simulink model "Elevator"  (R2023b)
settings: Solver=ode45  StartTime=0.0  StopTime=35  RelTol=1e-3
PreLoadFcn:
  | addpath(fullfile("ElevatorSupport","Scripts"));
  | addpath(fullfile("ElevatorSupport","Geometries"));
model workspace: external: MATLAB File Parameters.m (data not in the file)
undefined symbols (not defined in the file): BuildingTop, CabinFrame, CabinTopPlate, CounterWeight, CounterWeightFrame, CouterWeightRail, D, Door, DoorMechanismPlate, DoorPart, DoorStairOutTime1, DoorStairOutTime2, ElevatorCabin, ElevatorRail, Floor, FloorHeight, FloorStairOut, FloorTimeStairOut, g, K, MotorShaft, PrismaticJoint, Pulley, RevoluteJoint, RigidTransform, scale, Shaft, StairOutTime1, StairOutTime2, X, x, x2, Y, Z
libraries: sm_lib x283, nesl_utility x47
(part 1 of 6)
CloseFcn:
  | try
  |     close(fh);
  | catch
  | end
  | 
  | clear fh
  | clear logsoutElevator simlogElevator;
  | 
  | rmpath(fullfile("ElevatorSupport","Scripts"));
  | rmpath(fullfile("ElevatorSupport","Geometries"))
settings Model: Creator=The MathWorks, Inc.  LastModifiedBy=Aryasetya
settings SolverCC: AlgebraicLoopSolver=TrustRegion
settings DataIOCC: SaveTime=off  ReturnWorkspaceOutputs=off  SignalLoggingName=logsoutElevator
settings OptimizationCC: ReuseModelBlockBuffer=off
settings DebuggingCC: UnconnectedInputMsg=warning  UnconnectedOutputMsg=warning  UnconnectedLineMsg=warning  SubsystemReferenceDiagnosticForUnitTest=warning  SymbolicDimsDataTypeCodeGenerationDiagnostic=none
settings ModelReferenceCC: EnableRefExpFcnMdlSchedulingChecks=on
settings RTWCC: DLArmComputeVersion=19.05
settings SimscapeCC: SimscapeLogType=all  SimscapeLogSimulationStatistics=on  SimscapeLogName=simlogElevator  SimscapeLogLimitData=off
settings ExplorerConfigSet: InternalSimMechanicsExplorerSettings="<ExplorerConfiguration><canonicalview>default</canonicalview><AnimationSetting><BasePlaybackSpeed>1.0</BasePlaybackSpeed><PlaybackSpeedFactor>1.0</PlaybackSpeedFactor></AnimationSetting><TilePanel><TileInfo><Tiles Columns=\"2\" Count=\"2\" Rows=\"1\"><Column Weight=\"0.5\"/><Column Weight=\"0.5\"/><Row Weight=\"1\"/><Tile Height=\"1\" Width=\"1\" X=\"0\" Y=\"0\"/><Tile Height=\"1\" Width=\"1\" X=\"1\" Y=\"0\"/></Tiles></TileInfo><SceneInfo><SceneViewer><BGColor><R>1</R><G>1</G><B>1</B></BGColor><Camera><DoPerspective>off</DoPerspective><Position><X>20.7086531676557151</X><Y>-1.02984379292616524</Y><Z>-11.0864965005865486</Z></Position><Center><X>0.581530353759752927</X><Y>-1.02984379292616524</Y><Z>-11.0864965005865486</Z></Center><Up><X>-0</X><Y>0</Y><Z>1</Z></Up><ViewLimDist>1</ViewLimDist><YLim>16.4085643386840836</YLim><XLim>12.1235252438684942</XLim></Camera></SceneViewer><SceneViewer><BGColor><R>1</R><G>1</G><B>1</B></BGColor><Camera><DoPerspective>off</DoPerspective><Position><X>16.0519528198950141</X><Y>-9.70748669894142147</Y><Z>-4.07379558754266302</Z></Position><Center><X>-0.762288983658603869</X><Y>0.000137372139278557626</Y><Z>-12.8970022525360406</Z></Center><Up><X>-0.368402698741947754</X><Y>0.189189529780353194</Y><Z>0.910212488038446565</Z></Up><ViewLimDist>1</ViewLimDist><YLim>17.267396482909362</YLim><XLim>12.7580763822769807</XLim></Camera></SceneViewer></SceneInfo></TilePanel><MechEditorPanel><Cameras><Camera><Id>Camera1</Id><Value><Name>Camera1</Name><NativeCamera><PositionKeyframeSet><Keyframe><Time>+1.4390386105436841e+00</Time><Value><X>-1.9862962897423667e+01</X><Y>+3.7052197674734106e+00</Y><Z>+3.0536805221501222e+01</Z></Value></Keyframe><Keyframe><Time>+5.0767389598235519e+00</Time><Value><X>-4.7342144342170034e+00</X><Y>-1.0515849016541027e+01</Y><Z>+1.0916291278670778e+01</Z></Value></Keyframe><Keyframe><Time>+1.0381173794619109e+01</Time><Value><X>+1.3085629284472713e+00</X><Y>-1.0832577523234079e+01</Y><Z>+3.8731290903665652e+01</Z></Value></Keyframe><Keyframe><Time>+2.0000000000000000e+01</Time><Value><X>-1.9862962897423667e+01</X><Y>+3.7052197674734106e+00</Y><Z>+3.0536805221501222e+01</Z></Value></Keyframe></PositionKeyframeSet><CenterKeyframeSet><Keyframe><Time>+1.4390386105436841e+00</Time><Value><X>+2.3195990578990404e+00</X><Y>-1.1335086534382448e+01</Y><Z>+1.0722456628381920e+00</Z></Value></Keyframe><Keyframe><Time>+5.0767389598235519e+00</Time><Value><X>+1.2004004088622686e+00</X><Y>-1.4539659485468171e+01</Y><Z>+3.0334861791598531e+00</Z></Value></Keyframe><Keyframe><Time>+1.0381173794619109e+01</Time><Value><X>+1.3085629284472713e+00</X><Y>-1.0832577523234079e+01</Y><Z>+1.2891524079708603e+00</Z></Value></Keyframe><Keyframe><Time>+2.0000000000000000e+01</Time><Value><X>+2.3195990578990333e+00</X><Y>-1.1335086534382443e+01</Y><Z>+1.0722456628382027e+00</Z></Value></Keyframe></CenterKeyframeSet><UpVectorKeyframeSet><Keyframe><Time>+1.4390386105436841e+00</Time><Value><X>+2.1048840196857138e-01</X><Y>+9.2576466533046864e-01</Y><Z>-3.1409300702543935e-01</Z></Value></Keyframe><Keyframe><Time>+5.0767389598235519e+00</Time><Value><X>+2.1048840196857138e-01</X><Y>+9.2576466533046875e-01</Y><Z>-3.1409300702543930e-01</Z></Value></Keyframe><Keyframe><Time>+1.0381173794619109e+01</Time><Value><X>+0.0000000000000000e+00</X><Y>+1.0000000000000000e+00</Y><Z>-0.0000000000000000e+00</Z></Value></Keyframe><Keyframe><Time>+2.0000000000000000e+01</Time><Value><X>+2.1048840196857138e-01</X><Y>+9.2576466533046875e-01</Y><Z>-3.1409300702543935e-01</Z></Value></Keyframe></UpVectorKeyframeSet></NativeCamera></Value></Camera><Camera><Id>Camera2</Id><Value><Name>Camera2</Name><NativeCamera><PositionKeyframeSet/><CenterKeyframeSet/><UpVectorKeyframeSet/></NativeCamera></Value></Camera></Cameras><GfxPanelCameraMap/><VideoCreator><PlaybackSpeedRatio>1.0</PlaybackSpeedRatio><FrameRate>30</FrameRate><VideoFormat>Motion JPEG AVI</VideoFormat><FrameSize>auto</FrameSize></VideoCreator></MechEditorPanel></ExplorerConfiguration>"

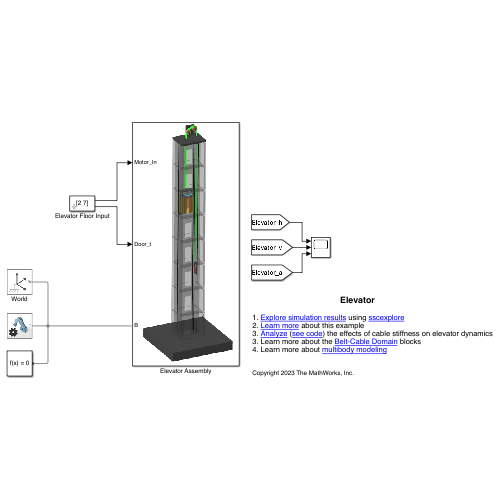
[thumbnail: Simulink's stored preview of the top-level diagram]
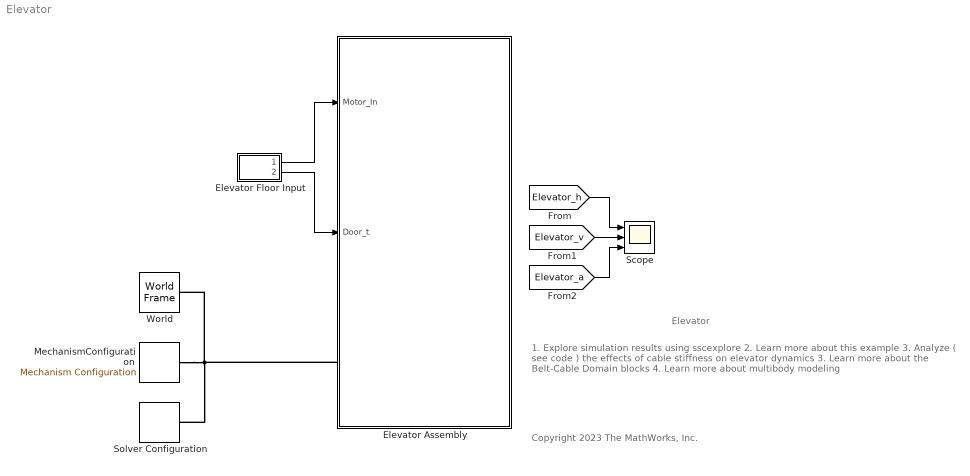
== system Elevator ==
  note: Copyright 2023 The MathWorks, Inc.
  note: 1. Explore simulation results using sscexplore
      | 2. Learn more about this example
      | 3. Analyze ( see code ) the effects of cable stiffness on elevator dynamics
      | 3. Learn more about the Belt-Cable Domain blocks
      | 4. Learn more about multibody modeling
  note: Elevator
  Elevator Assembly : Subsystem
      mask Display: image(fullfile('ElevatorSupport','Images','Full.png'));
  Elevator Floor Input : Subsystem  mask(Elevator Floors Input){FloorNums=[2 7]}
      mask prompts: FloorNums "Enter Floor Numbers"
      mask help:
      | Provide the floor numbers (1 to 7) for the elevator. This should be a (1 x n) vector. (n<=3)
      |
      | For example, an input of [4 2] means the elevator will go to the 4th Floor first and then the 2nd Floor.
      mask init:
      | if ~isrow(str2num(get_param(gcb,'FloorNums')))
      |     error('Input should be a row vector');
      | end
      | 
      | if length(str2num(get_param(gcb,'FloorNums')))>3
      |     error('Length of input row vector should not be greater then 3');
      | end
      | 
      | if any(str2num(get_param(gcb,'FloorNums'))>7)
      |     error('Elevator can not go above 7 floors for this system');
      | end
      | 
      | if any(str2num(get_param(gcb,'FloorNums'))<=0)
      |     error('Elevator floor input should be greater then 0');
      | end
      mask Display: disp(get_param(gcb,'FloorNums'));
  MechanismConfiguration : sm_lib/Utilities/Mechanism Configuration  UniformGravity=Constant  GravityVector=[0 0 -g]  GravityVectorUnits=m/s^2  LinearizationDelta=0.001  JointModeTransitionNonlinearIterations=2
  Scope : Scope  NumInputPorts=3
  Solver Configuration : nesl_utility/Solver Configuration  PhysicalDomain=network_engine_domain  SubClassName=solver  LeftPortType=input  RightPortType=generic  Tones=[]  Harmonics=[]  SimulateNoise=off  Profile=off  UseLocalSampling=off  EnableSwitchedLinearOptims=on  FrequencyDomain=off  UseCCode=off  RelTol=0.001  AbsTol=1e-06  MinStep=1e-09  ToWorkspace=off  RevertToSquareIcSolve=off  NumHomotopyIterations=100  PhasorMode=off  PhasorModeNumHarmonics=1  ConsistencySolver=NEWTON_FTOL  IndexReductionMethod=DerivativeReplacement  DoDC=off  ResidualTolerance=1e-09  ConsistencyTolSource=GLOBAL  ConsistencyAbsTol=0.001  ConsistencyRelTol=0.001  ConsistencyTolFactor=0.001  UseLocalSolver=off  LocalSolverChoice=NE_BACKWARD_EULER_ADVANCER  ResolveIndetEquations=on  FunctionEvalNumThread=1  LocalSolverSampleTime=0.001  DoFixedCost=off  MaxNonlinIter=3  MaxModeIter=2  ComputeImpulses=off  ImpulseIterations=1  LinearAlgebra=auto  LinearAlgebraNumThread=0  EquationFormulation=NE_TIME_EF  DelaysMemoryBudget=1024  AutomaticFiltering=on  FilteringTimeConstant=0.001  PartitionStorageMethod=AS_NEEDED  PartitionMemoryBudget=1024  PartitionMethod=ROBUST  MultibodyUseLocalSolver=off  MultibodyLocalSolverChoice=ODE1  MultibodyLocalSolverSampleTime=0.001
  World : sm_lib/Frames and Transforms/World Frame
  wires:
  Elevator Floor Input/1(MotorMotion) -> Elevator Assembly/1(Motor_In)
  Elevator Floor Input/2(DoorOperationTimes) -> Elevator Assembly/2(Door_t)
  [Elevator_h] -> Scope/1
  [Elevator_v] -> Scope/2
  [Elevator_a] -> Scope/3
  connections:
  MechanismConfiguration/RConn1 -- World/RConn1 -- Elevator Assembly/LConn1 -- Solver Configuration/RConn1

== system Elevator/Elevator Assembly ==
  Motor_In : Inport
  Door_t : Inport  Port=2
  Building : Subsystem
      mask Display: image(fullfile('ElevatorSupport','Images','Building.png'));
  CounterWeight : Subsystem
      mask Display: image(fullfile('ElevatorSupport','Images','CounterWeight.png'));
  CounterWeightPrismatic : Subsystem
  ElevatorCabin : Subsystem
      mask Display: image(fullfile('ElevatorSupport','Images','Cabin.png'));
  ElevatorPrismatic : Subsystem
  MotorPulley : Subsystem
      mask Display: image(fullfile('ElevatorSupport','Images','MotorPulley.png'));
  Rigid Transform : sm_lib/Frames and Transforms/Rigid Transform  TranslationMethod=None  TranslationStandardOffset=0  TranslationStandardOffsetUnits=m  TranslationStandardAxis=+Z  TranslationCartesianOffset=[0 0 0]  TranslationCartesianOffsetUnits=m  TranslationROffset=0  TranslationROffsetUnits=m  TranslationZOffset=0  TranslationZOffsetUnits=m  TranslationThetaOffset=0  TranslationThetaOffsetUnits=deg  RotationMethod=StandardAxis  RotationAngleUnits=deg  RotationStandardAxis=+Z  RotationAngle=-90  RotationArbitraryAxis=[0 0 1]  FollAlignAxisA=+Y  BaseAlignAxisA=-Y  FollAlignAxisB=+X  BaseAlignAxisB=-X  RotationSequenceAxes=FollowerAxes  RotationSequence=XYX  RotationSequenceAngles=[0 0 0]  RotationSequenceAnglesUnits=deg  RotationMatrix=[1 0 0; 0 1 0; 0 0 1]  Quaternion=[1 0 0 0]
  B : PMIOPort  Side=Left
  wires:
  Door_t/1 -> ElevatorCabin/1(door_t)
  ElevatorPrismatic/1(pos) -> ElevatorCabin/2(h)
  Motor_In/1 -> MotorPulley/1(Motor_In)
  connections:
  MotorPulley/RConn1 -- ElevatorCabin/LConn5
  MotorPulley/RConn6 -- CounterWeight/RConn5
  CounterWeight/RConn3 -- MotorPulley/RConn4
  Rigid Transform/LConn1 -- B/RConn1
  MotorPulley/RConn7 -- ElevatorCabin/LConn1
  MotorPulley/RConn10 -- ElevatorCabin/LConn4
  MotorPulley/RConn5 -- CounterWeight/RConn4
  ElevatorPrismatic/LConn1 -- Building/LConn2
  CounterWeight/LConn1 -- CounterWeightPrismatic/RConn1
  CounterWeight/RConn2 -- MotorPulley/RConn3
  MotorPulley/RConn9 -- ElevatorCabin/LConn3
  Building/LConn1 -- MotorPulley/LConn1
  MotorPulley/RConn2 -- CounterWeight/RConn1
  MotorPulley/RConn8 -- ElevatorCabin/LConn2
  ElevatorPrismatic/RConn1 -- ElevatorCabin/RConn1
  Building/RConn1 -- Rigid Transform/RConn1
  CounterWeightPrismatic/LConn1 -- Building/LConn3

== system Elevator/Elevator Floor Input ==
  Abs : Abs  SaturateOnIntegerOverflow=off
  Clock1 : Clock
  Clock3 : Clock
  Constant1 : Constant
  Constant2 : Constant  Value=1.5
  FloorChangesStairSignal : Subsystem  mask{FloorNums=FloorNums}
      mask prompts: FloorNums "Enter Floor Nums for Elevator"
      mask init:
      | [FloorStairOut,FloorTimeStairOut,StairOutTime1,StairOutTime2,DoorStairOutTime1,DoorStairOutTime2]...
      |  = getLookUpTableData(FloorNums);
  Gain : Gain  Gain=1/Pulley.radius
  Gain1 : Gain  Gain=FloorHeight
  Integrator1 : Integrator
  MATLAB Function : MATLAB Function  TreatAsAtomicUnit=on
  MotorDirection : Signum
  Product : Product
  Scope1 : Scope
  MotorMotion : Outport  VectorParamsAs1DForOutWhenUnconnected=off
  DoorOperationTimes : Outport  Port=2  VectorParamsAs1DForOutWhenUnconnected=off
  wires:
  FloorChangesStairSignal/3(DoorTimeChanges) -> DoorOperationTimes/1
  Abs/1 -> MATLAB Function/2(total_dis)
  FloorChangesStairSignal/1(FloorChanges) -> MotorDirection/1, Gain1/1
  FloorChangesStairSignal/2(TimeChanges) -> MATLAB Function/5(StepTime)
  Clock1/1 -> FloorChangesStairSignal/1(In1)
  MATLAB Function/1(v_t) -> Product/2
  Product/1 -> Integrator1/1
  MotorDirection/1 -> Product/1
  Gain/1 -> MotorMotion/1
  Gain1/1 -> Abs/1
  Clock3/1 -> MATLAB Function/1(t)
  Constant1/1 -> MATLAB Function/3(a)
  Constant2/1 -> MATLAB Function/4(v_const)
  Integrator1/1 -> Scope1/1, Gain/1

== system Elevator/Elevator Assembly/Building ==
  Floors : Subsystem
      mask Display: image(fullfile('ElevatorSupport','Images','Floor.png'));
  LongRail_1_RIGID : Subsystem
      mask Display: image(fullfile('ElevatorSupport','Images','Rails.png'));
  LongRail_2_RIGID : Subsystem
      mask Display: image(fullfile('ElevatorSupport','Images','Rails.png'));
  Planar : sm_lib/Joints/Planar Joint  JointMode=Normal  SenseConstraintForce=off  SenseConstraintForceX=off  SenseConstraintForceY=off  SenseConstraintForceZ=off  SenseConstraintTorque=off  SenseConstraintTorqueX=off  SenseConstraintTorqueY=off  SenseConstraintTorqueZ=off  SenseTotalForce=off  SenseTotalForceX=off  SenseTotalForceY=off  SenseTotalForceZ=off  SenseTotalTorque=off  SenseTotalTorqueX=off  SenseTotalTorqueY=off  SenseTotalTorqueZ=off  CompositeWrenchDir=FollowerOnBase  CompositeWrenchFrame=BaseFrame  PxEquilibriumPosition=0  PxEquilibriumPositionUnits=m  PxSpringStiffness=0  PxSpringStiffnessUnits=N/m  PxDampingCoefficient=0  PxDampingCoefficientUnits=N/(m/s)  PxTorqueActuationMode=NoTorque  PxMotionActuationMode=ComputedMotion  PxSensePosition=off  PxSenseVelocity=off  PxSenseAcceleration=off  PxSenseTorqueForce=off  PxSenseLowerLimitTorqueForce=off  PxSenseUpperLimitTorqueForce=off  PxLowerLimitSpecify=off  PxLowerLimitBound=-1  PxLowerLimitBoundUnits=m  PxLowerLimitStiffness=1e6  PxLowerLimitStiffnessUnits=N/m  PxLowerLimitDamping=1e3  PxLowerLimitDampingUnits=N/(m/s)  PxLowerLimitTransitionRegionWidth=1e-4  PxLowerLimitTransitionRegionWidthUnits=m  PxUpperLimitSpecify=off  PxUpperLimitBound=1  PxUpperLimitBoundUnits=m  PxUpperLimitStiffness=1e6  PxUpperLimitStiffnessUnits=N/m  PxUpperLimitDamping=1e3  PxUpperLimitDampingUnits=N/(m/s)  PxUpperLimitTransitionRegionWidth=1e-4  PxUpperLimitTransitionRegionWidthUnits=m  PxPositionTargetSpecify=off  PxPositionTargetPriority=High  PxPositionTargetValue=0  PxPositionTargetValueUnits=m  PxVelocityTargetSpecify=off  PxVelocityTargetPriority=High  PxVelocityTargetValue=0  PxVelocityTargetValueUnits=m/s  PyEquilibriumPosition=0  PyEquilibriumPositionUnits=m  PySpringStiffness=0  PySpringStiffnessUnits=N/m  PyDampingCoefficient=0  PyDampingCoefficientUnits=N/(m/s)  PyTorqueActuationMode=NoTorque  PyMotionActuationMode=ComputedMotion  PySensePosition=off  PySenseVelocity=off  PySenseAcceleration=off  PySenseTorqueForce=off  PySenseLowerLimitTorqueForce=off  PySenseUpperLimitTorqueForce=off  PyLowerLimitSpecify=off  PyLowerLimitBound=-1  PyLowerLimitBoundUnits=m  PyLowerLimitStiffness=1e6  PyLowerLimitStiffnessUnits=N/m  PyLowerLimitDamping=1e3  PyLowerLimitDampingUnits=N/(m/s)  PyLowerLimitTransitionRegionWidth=1e-4  PyLowerLimitTransitionRegionWidthUnits=m  PyUpperLimitSpecify=off  PyUpperLimitBound=1  PyUpperLimitBoundUnits=m  PyUpperLimitStiffness=1e6  PyUpperLimitStiffnessUnits=N/m  PyUpperLimitDamping=1e3  PyUpperLimitDampingUnits=N/(m/s)  PyUpperLimitTransitionRegionWidth=1e-4  PyUpperLimitTransitionRegionWidthUnits=m  PyPositionTargetSpecify=off  PyPositionTargetPriority=High  PyPositionTargetValue=0  PyPositionTargetValueUnits=m  PyVelocityTargetSpecify=off  PyVelocityTargetPriority=High  PyVelocityTargetValue=0  PyVelocityTargetValueUnits=m/s  RzEquilibriumPosition=0  RzEquilibriumPositionUnits=rad  RzSpringStiffness=0  RzSpringStiffnessUnits=N*m/rad  RzDampingCoefficient=0  RzDampingCoefficientUnits=N*m/(rad/s)  RzTorqueActuationMode=NoTorque  RzMotionActuationMode=ComputedMotion  RzSensePosition=off  RzSenseVelocity=off  RzSenseAcceleration=off  RzSenseTorqueForce=off  RzSenseLowerLimitTorqueForce=off  RzSenseUpperLimitTorqueForce=off  RzLowerLimitSpecify=off  RzLowerLimitBound=-90  RzLowerLimitBoundUnits=deg  RzLowerLimitStiffness=1e4  RzLowerLimitStiffnessUnits=N*m/deg  RzLowerLimitDamping=10  RzLowerLimitDampingUnits=N*m/(deg/s)  RzLowerLimitTransitionRegionWidth=0.1  RzLowerLimitTransitionRegionWidthUnits=deg  RzUpperLimitSpecify=off  RzUpperLimitBound=90  RzUpperLimitBoundUnits=deg  RzUpperLimitStiffness=1e4  RzUpperLimitStiffnessUnits=N*m/deg  RzUpperLimitDamping=10  RzUpperLimitDampingUnits=N*m/(deg/s)  RzUpperLimitTransitionRegionWidth=0.1  RzUpperLimitTransitionRegionWidthUnits=deg  RzPositionTargetSpecify=off  RzPositionTargetPriority=High  RzPositionTargetValue=0  RzPositionTargetValueUnits=deg  RzVelocityTargetSpecify=off  RzVelocityTargetPriority=High  RzVelocityTargetValue=0  RzVelocityTargetValueUnits=deg/s
  Prismatic : sm_lib/Joints/Prismatic Joint  JointMode=Normal  SenseConstraintForce=off  SenseConstraintForceX=off  SenseConstraintForceY=off  SenseConstraintForceZ=off  SenseConstraintTorque=off  SenseConstraintTorqueX=off  SenseConstraintTorqueY=off  SenseConstraintTorqueZ=off  SenseTotalForce=off  SenseTotalForceX=off  SenseTotalForceY=off  SenseTotalForceZ=off  SenseTotalTorque=off  SenseTotalTorqueX=off  SenseTotalTorqueY=off  SenseTotalTorqueZ=off  CompositeWrenchDir=FollowerOnBase  CompositeWrenchFrame=BaseFrame  EquilibriumPosition=0  EquilibriumPositionUnits=m  SpringStiffness=0  SpringStiffnessUnits=N/m  DampingCoefficient=0  DampingCoefficientUnits=N/(m/s)  TorqueActuationMode=NoTorque  MotionActuationMode=ComputedMotion  SensePosition=off  SenseVelocity=off  SenseAcceleration=off  SenseTorqueForce=off  SenseLowerLimitTorqueForce=off  SenseUpperLimitTorqueForce=off  LowerLimitSpecify=off  LowerLimitBound=-1  LowerLimitBoundUnits=m  LowerLimitStiffness=1e6  LowerLimitStiffnessUnits=N/m  LowerLimitDamping=1e3  LowerLimitDampingUnits=N/(m/s)  LowerLimitTransitionRegionWidth=1e-4  LowerLimitTransitionRegionWidthUnits=m  UpperLimitSpecify=off  UpperLimitBound=1  UpperLimitBoundUnits=m  UpperLimitStiffness=1e6  UpperLimitStiffnessUnits=N/m  UpperLimitDamping=1e3  UpperLimitDampingUnits=N/(m/s)  UpperLimitTransitionRegionWidth=1e-4  UpperLimitTransitionRegionWidthUnits=m  PositionTargetSpecify=on  PositionTargetPriority=Low  PositionTargetValue=PrismaticJoint(1).Pz.Pos  PositionTargetValueUnits=m  VelocityTargetSpecify=off  VelocityTargetPriority=High  VelocityTargetValue=0  VelocityTargetValueUnits=m/s
  Rail1 : Subsystem
      mask Display: image(fullfile('ElevatorSupport','Images','Rails.png'));
  Rail2 : Subsystem
      mask Display: image(fullfile('ElevatorSupport','Images','Rails.png'));
  F1 : PMIOPort  Side=Left
  B : PMIOPort  Port=2  Side=Right
  F2 : PMIOPort  Port=3  Side=Left
  F3 : PMIOPort  Port=4  Side=Left
  connections:
  Rail1/LConn2 -- Rail2/RConn1
  Rail1/LConn1 -- B/RConn1
  LongRail_1_RIGID/LConn2 -- LongRail_2_RIGID/LConn2
  Floors/RConn1 -- Rail2/LConn1
  Rail1/RConn1 -- Planar/LConn1
  LongRail_2_RIGID/LConn1 -- Planar/RConn1
  Rail1/RConn2 -- Prismatic/LConn1
  LongRail_1_RIGID/LConn3 -- Prismatic/RConn1
  F2/RConn1 -- Rail2/LConn2
  Floors/LConn1 -- F1/RConn1
  LongRail_1_RIGID/LConn1 -- F3/RConn1

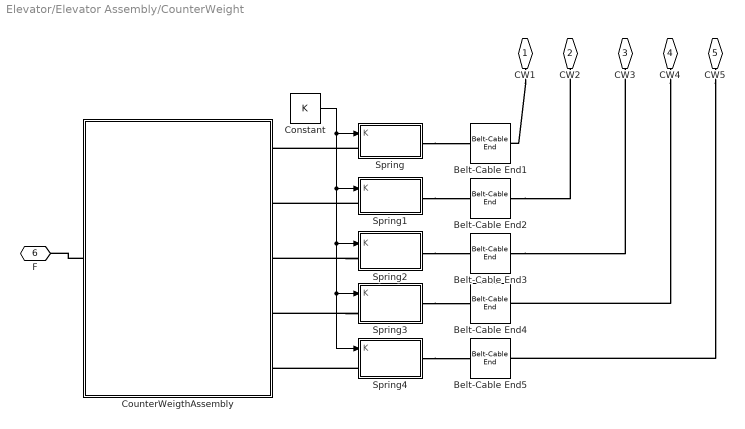
== system Elevator/Elevator Assembly/CounterWeight ==
  Belt-Cable End{1..5} (5 alike) : sm_lib/Belts and Cables/Belt-Cable End
  Constant : Constant  Value=K
  CounterWeigthAssembly : Subsystem
      mask Display: image(fullfile('ElevatorSupport','Images','CounterWeight.png'));
  Spring : Subsystem
  Spring1 : Subsystem
  Spring2 : Subsystem
  Spring3 : Subsystem
  Spring4 : Subsystem
  CW1 : PMIOPort  Side=Right
  CW2 : PMIOPort  Port=2  Side=Right
  CW3 : PMIOPort  Port=3  Side=Right
  CW4 : PMIOPort  Port=4  Side=Right
  CW5 : PMIOPort  Port=5  Side=Right
  F : PMIOPort  Port=6  Side=Left
  wires:
  Constant/1 -> Spring/1(K), Spring1/1(K), Spring2/1(K), Spring3/1(K), Spring4/1(K)
  connections:
  Spring3/RConn1 -- Belt-Cable End4/LConn1
  Spring2/RConn1 -- Belt-Cable End3/LConn1
  Spring2/LConn1 -- CounterWeigthAssembly/RConn3
  Spring4/LConn1 -- CounterWeigthAssembly/RConn5
  Spring/LConn1 -- CounterWeigthAssembly/RConn1
  Belt-Cable End2/RConn1 -- CW2/RConn1
  Spring1/LConn1 -- CounterWeigthAssembly/RConn2
  Spring1/RConn1 -- Belt-Cable End2/LConn1
  Belt-Cable End3/RConn1 -- CW3/RConn1
  CW1/RConn1 -- Belt-Cable End1/RConn1
  Spring4/RConn1 -- Belt-Cable End5/LConn1
  Spring3/LConn1 -- CounterWeigthAssembly/RConn4
  Spring/RConn1 -- Belt-Cable End1/LConn1
  CounterWeigthAssembly/LConn1 -- F/RConn1
  CW5/RConn1 -- Belt-Cable End5/RConn1
  CW4/RConn1 -- Belt-Cable End4/RConn1

== system Elevator/Elevator Assembly/CounterWeightPrismatic ==
  Prismatic Joint : sm_lib/Joints/Prismatic Joint  JointMode=Normal  SenseConstraintForce=off  SenseConstraintForceX=off  SenseConstraintForceY=off  SenseConstraintForceZ=off  SenseConstraintTorque=off  SenseConstraintTorqueX=off  SenseConstraintTorqueY=off  SenseConstraintTorqueZ=off  SenseTotalForce=off  SenseTotalForceX=off  SenseTotalForceY=off  SenseTotalForceZ=off  SenseTotalTorque=off  SenseTotalTorqueX=off  SenseTotalTorqueY=off  SenseTotalTorqueZ=off  CompositeWrenchDir=FollowerOnBase  CompositeWrenchFrame=BaseFrame  EquilibriumPosition=0  EquilibriumPositionUnits=m  SpringStiffness=0  SpringStiffnessUnits=N/m  DampingCoefficient=0  DampingCoefficientUnits=N/(m/s)  TorqueActuationMode=NoTorque  MotionActuationMode=ComputedMotion  SensePosition=off  SenseVelocity=off  SenseAcceleration=off  SenseTorqueForce=off  SenseLowerLimitTorqueForce=off  SenseUpperLimitTorqueForce=off  LowerLimitSpecify=off  LowerLimitBound=-1  LowerLimitBoundUnits=m  LowerLimitStiffness=1e6  LowerLimitStiffnessUnits=N/m  LowerLimitDamping=1e3  LowerLimitDampingUnits=N/(m/s)  LowerLimitTransitionRegionWidth=1e-4  LowerLimitTransitionRegionWidthUnits=m  UpperLimitSpecify=off  UpperLimitBound=1  UpperLimitBoundUnits=m  UpperLimitStiffness=1e6  UpperLimitStiffnessUnits=N/m  UpperLimitDamping=1e3  UpperLimitDampingUnits=N/(m/s)  UpperLimitTransitionRegionWidth=1e-4  UpperLimitTransitionRegionWidthUnits=m  PositionTargetSpecify=on  PositionTargetPriority=High  PositionTargetValue=7.5  PositionTargetValueUnits=m  VelocityTargetSpecify=off  VelocityTargetPriority=High  VelocityTargetValue=0  VelocityTargetValueUnits=m/s
  Rigid Transform : sm_lib/Frames and Transforms/Rigid Transform  TranslationMethod=None  TranslationStandardOffset=0  TranslationStandardOffsetUnits=m  TranslationStandardAxis=+Z  TranslationCartesianOffset=[0 0 0]  TranslationCartesianOffsetUnits=m  TranslationROffset=0  TranslationROffsetUnits=m  TranslationZOffset=0  TranslationZOffsetUnits=m  TranslationThetaOffset=0  TranslationThetaOffsetUnits=deg  RotationMethod=StandardAxis  RotationAngleUnits=deg  RotationStandardAxis=+Y  RotationAngle=90  RotationArbitraryAxis=[0 0 1]  FollAlignAxisA=+X  BaseAlignAxisA=+Y  FollAlignAxisB=+Y  BaseAlignAxisB=+Z  RotationSequenceAxes=FollowerAxes  RotationSequence=XYX  RotationSequenceAngles=[0 0 0]  RotationSequenceAnglesUnits=deg  RotationMatrix=[1 0 0; 0 1 0; 0 0 1]  Quaternion=[1 0 0 0]
  Rigid Transform1 : sm_lib/Frames and Transforms/Rigid Transform  TranslationMethod=None  TranslationStandardOffset=0  TranslationStandardOffsetUnits=m  TranslationStandardAxis=+Z  TranslationCartesianOffset=[0 0 0]  TranslationCartesianOffsetUnits=m  TranslationROffset=0  TranslationROffsetUnits=m  TranslationZOffset=0  TranslationZOffsetUnits=m  TranslationThetaOffset=0  TranslationThetaOffsetUnits=deg  RotationMethod=StandardAxis  RotationAngleUnits=deg  RotationStandardAxis=+Y  RotationAngle=-90  RotationArbitraryAxis=[0 0 1]  FollAlignAxisA=+X  BaseAlignAxisA=+Y  FollAlignAxisB=+Y  BaseAlignAxisB=+Z  RotationSequenceAxes=FollowerAxes  RotationSequence=XYX  RotationSequenceAngles=[0 0 0]  RotationSequenceAnglesUnits=deg  RotationMatrix=[1 0 0; 0 1 0; 0 0 1]  Quaternion=[1 0 0 0]
  B : PMIOPort  Side=Left
  F : PMIOPort  Port=2  Side=Right
  connections:
  Prismatic Joint/LConn1 -- Rigid Transform/RConn1
  Prismatic Joint/RConn1 -- Rigid Transform1/LConn1
  Rigid Transform1/RConn1 -- F/RConn1
  Rigid Transform/LConn1 -- B/RConn1

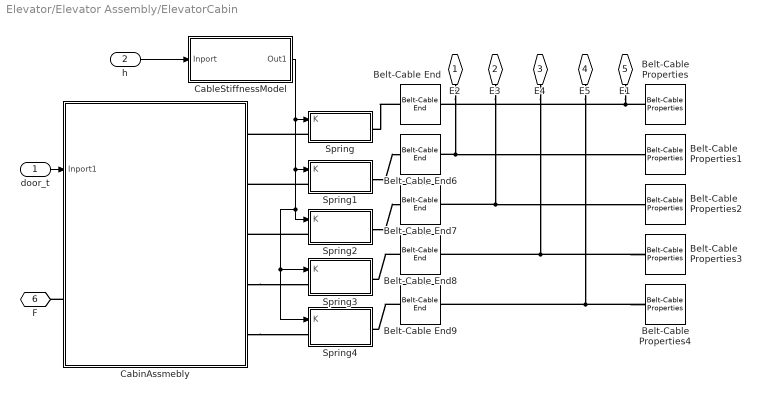
== system Elevator/Elevator Assembly/ElevatorCabin ==
  door_t : Inport
  h : Inport  Port=2
  Belt-Cable Properties{,1..4} (5 alike) : sm_lib/Belts and Cables/Belt-Cable Properties  DrumBeltCableAlignment=Unrestricted  GraphicType=PitchLine  GraphicVisPropType=SimpleVisualProperties  GraphicDiffuseColor=[0.2 1.0 0.2]  GraphicSpecularColor=[0.5 0.5 0.5 1.0]  GraphicAmbientColor=[0.15 0.15 0.15 1.0]  GraphicEmissiveColor=[0.0 0.0 0.0 1.0]  GraphicShininess=75  GraphicOpacity=1.0
  Belt-Cable End{,6..9} (5 alike) : sm_lib/Belts and Cables/Belt-Cable End
  CabinAssmebly : Subsystem
      mask Display: image(fullfile('ElevatorSupport','Images','CabinAssembly.png'));
  CableStiffnessModel : Subsystem  mask(Cable Stiffness){StiffnessModelChoice=Constant Stiffness}
      mask prompts: StiffnessModelChoice "StiffnessModel"
      mask help: Select Constant or Variable Stiffness values for approximating cable stiffness.
      mask TypeOptions StiffnessModelChoice: Constant Stiffness | Variable Stiffness
      mask Display: disp(get_param(gcb,'StiffnessModelChoice'))
  Spring : Subsystem
  Spring1 : Subsystem
  Spring2 : Subsystem
  Spring3 : Subsystem
  Spring4 : Subsystem
  E2 : PMIOPort  Side=Left
  E3 : PMIOPort  Port=2  Side=Left
  E4 : PMIOPort  Port=3  Side=Left
  E5 : PMIOPort  Port=4  Side=Left
  E1 : PMIOPort  Port=5  Side=Left
  F : PMIOPort  Port=6  Side=Right
  wires:
  door_t/1 -> CabinAssmebly/1(Inport1)
  CableStiffnessModel/1(Out1) -> Spring1/1(K), Spring4/1(K), Spring3/1(K), Spring2/1(K), Spring/1(K)
  h/1 -> CableStiffnessModel/1(Inport)
  connections:
  Belt-Cable Properties4/LConn1 -- Belt-Cable End9/RConn1 -- E5/RConn1
  CabinAssmebly/RConn5 -- Spring4/LConn1
  E3/RConn1 -- Belt-Cable End7/RConn1 -- Belt-Cable Properties2/LConn1
  Belt-Cable Properties3/LConn1 -- Belt-Cable End8/RConn1 -- E4/RConn1
  Spring2/RConn1 -- Belt-Cable End7/LConn1
  E2/RConn1 -- Belt-Cable Properties1/LConn1 -- Belt-Cable End6/RConn1
  Spring/LConn1 -- CabinAssmebly/RConn1
  Belt-Cable End8/LConn1 -- Spring3/RConn1
  Belt-Cable End/LConn1 -- Spring/RConn1
  Spring2/LConn1 -- CabinAssmebly/RConn3
  Belt-Cable End9/LConn1 -- Spring4/RConn1
  Spring1/LConn1 -- CabinAssmebly/RConn2
  Spring1/RConn1 -- Belt-Cable End6/LConn1
  CabinAssmebly/RConn4 -- Spring3/LConn1
  CabinAssmebly/LConn1 -- F/RConn1
  E1/RConn1 -- Belt-Cable Properties/LConn1 -- Belt-Cable End/RConn1

== system Elevator/Elevator Assembly/ElevatorPrismatic ==
  Abs : Abs  SaturateOnIntegerOverflow=off
  Add : Sum  Inputs=+-
  Constant : Constant  Value=-25.25
  PS-Simulink Converter : nesl_utility/PS-Simulink Converter  PhysicalDomain=network_engine_domain  SubClassName=ps_output  LeftPortType=input  RightPortType=output  PseudoPeriodic=off  Frequencies=[]  VectorFormat=1-D array  Unit=inherit  AffineConversion=off
  PS-Simulink Converter1 : nesl_utility/PS-Simulink Converter  PhysicalDomain=network_engine_domain  SubClassName=ps_output  LeftPortType=input  RightPortType=output  PseudoPeriodic=off  Frequencies=[]  VectorFormat=1-D array  Unit=inherit  AffineConversion=off
  PS-Simulink Converter2 : nesl_utility/PS-Simulink Converter  PhysicalDomain=network_engine_domain  SubClassName=ps_output  LeftPortType=input  RightPortType=output  PseudoPeriodic=off  Frequencies=[]  VectorFormat=1-D array  Unit=inherit  AffineConversion=off
  Prismatic Joint : sm_lib/Joints/Prismatic Joint  JointMode=Normal  SenseConstraintForce=off  SenseConstraintForceX=off  SenseConstraintForceY=off  SenseConstraintForceZ=off  SenseConstraintTorque=off  SenseConstraintTorqueX=off  SenseConstraintTorqueY=off  SenseConstraintTorqueZ=off  SenseTotalForce=off  SenseTotalForceX=off  SenseTotalForceY=off  SenseTotalForceZ=off  SenseTotalTorque=off  SenseTotalTorqueX=off  SenseTotalTorqueY=off  SenseTotalTorqueZ=off  CompositeWrenchDir=FollowerOnBase  CompositeWrenchFrame=BaseFrame  EquilibriumPosition=0  EquilibriumPositionUnits=m  SpringStiffness=0  SpringStiffnessUnits=N/m  DampingCoefficient=0  DampingCoefficientUnits=N/(m/s)  TorqueActuationMode=NoTorque  MotionActuationMode=ComputedMotion  SensePosition=on  SenseVelocity=on  SenseAcceleration=on  SenseTorqueForce=off  SenseLowerLimitTorqueForce=off  SenseUpperLimitTorqueForce=off  LowerLimitSpecify=off  LowerLimitBound=-1  LowerLimitBoundUnits=m  LowerLimitStiffness=1e6  LowerLimitStiffnessUnits=N/m  LowerLimitDamping=1e3  LowerLimitDampingUnits=N/(m/s)  LowerLimitTransitionRegionWidth=1e-4  LowerLimitTransitionRegionWidthUnits=m  UpperLimitSpecify=off  UpperLimitBound=1  UpperLimitBoundUnits=m  UpperLimitStiffness=1e6  UpperLimitStiffnessUnits=N/m  UpperLimitDamping=1e3  UpperLimitDampingUnits=N/(m/s)  UpperLimitTransitionRegionWidth=1e-4  UpperLimitTransitionRegionWidthUnits=m  PositionTargetSpecify=on  PositionTargetPriority=High  PositionTargetValue=-25.25  PositionTargetValueUnits=m  VelocityTargetSpecify=off  VelocityTargetPriority=Low  VelocityTargetValue=10  VelocityTargetValueUnits=m/s
  Rigid Transform : sm_lib/Frames and Transforms/Rigid Transform  TranslationMethod=None  TranslationStandardOffset=0  TranslationStandardOffsetUnits=m  TranslationStandardAxis=+Z  TranslationCartesianOffset=[0 0 0]  TranslationCartesianOffsetUnits=m  TranslationROffset=0  TranslationROffsetUnits=m  TranslationZOffset=0  TranslationZOffsetUnits=m  TranslationThetaOffset=0  TranslationThetaOffsetUnits=deg  RotationMethod=StandardAxis  RotationAngleUnits=deg  RotationStandardAxis=+Y  RotationAngle=90  RotationArbitraryAxis=[0 0 1]  FollAlignAxisA=+X  BaseAlignAxisA=+Y  FollAlignAxisB=+Y  BaseAlignAxisB=+Z  RotationSequenceAxes=FollowerAxes  RotationSequence=XYX  RotationSequenceAngles=[0 0 0]  RotationSequenceAnglesUnits=deg  RotationMatrix=[1 0 0; 0 1 0; 0 0 1]  Quaternion=[1 0 0 0]
  Rigid Transform1 : sm_lib/Frames and Transforms/Rigid Transform  TranslationMethod=None  TranslationStandardOffset=0  TranslationStandardOffsetUnits=m  TranslationStandardAxis=+Z  TranslationCartesianOffset=[0 0 0]  TranslationCartesianOffsetUnits=m  TranslationROffset=0  TranslationROffsetUnits=m  TranslationZOffset=0  TranslationZOffsetUnits=m  TranslationThetaOffset=0  TranslationThetaOffsetUnits=deg  RotationMethod=StandardAxis  RotationAngleUnits=deg  RotationStandardAxis=+Y  RotationAngle=-90  RotationArbitraryAxis=[0 0 1]  FollAlignAxisA=+X  BaseAlignAxisA=+Y  FollAlignAxisB=+Y  BaseAlignAxisB=+Z  RotationSequenceAxes=FollowerAxes  RotationSequence=XYX  RotationSequenceAngles=[0 0 0]  RotationSequenceAnglesUnits=deg  RotationMatrix=[1 0 0; 0 1 0; 0 0 1]  Quaternion=[1 0 0 0]
  F : PMIOPort  Side=Right
  B : PMIOPort  Port=2  Side=Left
  pos : Outport  VectorParamsAs1DForOutWhenUnconnected=off
  tag scope: Elevator_a=global, Elevator_h=global, Elevator_v=global
  wires:
  PS-Simulink Converter/1 -> Add/2, pos/1
  Add/1 -> Abs/1
  Constant/1 -> Add/1
  PS-Simulink Converter2/1 -> [Elevator_v]  "v"
  PS-Simulink Converter1/1 -> [Elevator_a]  "a"
  Abs/1 -> [Elevator_h]  "h"
  connections:
  Prismatic Joint/LConn1 -- Rigid Transform/RConn1
  Prismatic Joint/RConn1 -- Rigid Transform1/LConn1
  PS-Simulink Converter/LConn1 -- Prismatic Joint/RConn2
  Rigid Transform1/RConn1 -- F/RConn1
  Rigid Transform/LConn1 -- B/RConn1
  PS-Simulink Converter1/LConn1 -- Prismatic Joint/RConn4
  PS-Simulink Converter2/LConn1 -- Prismatic Joint/RConn3

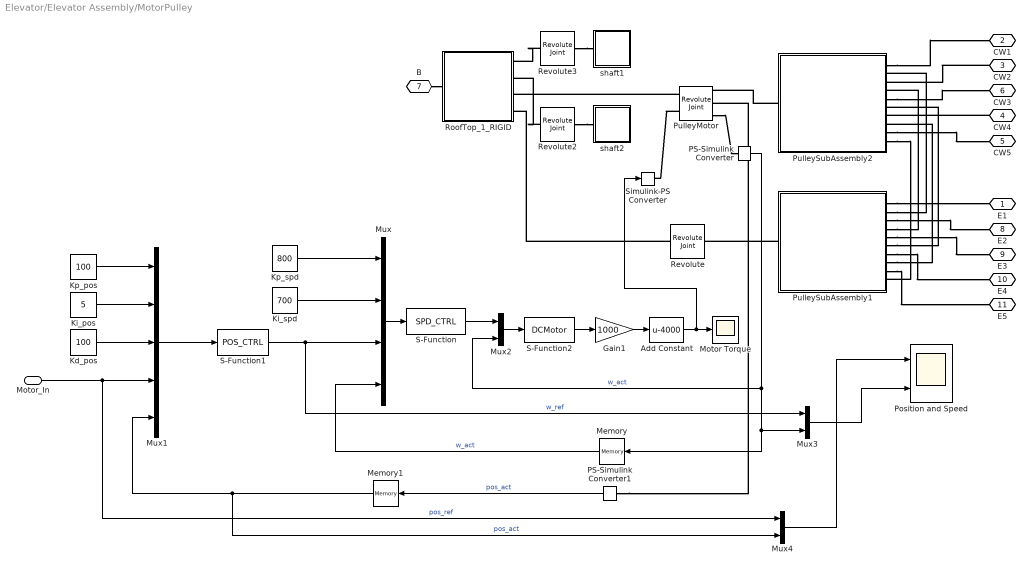
== system Elevator/Elevator Assembly/MotorPulley ==
  Motor_In : Inport
  Add Constant : Bias  Bias=-4000  SaturateOnIntegerOverflow=off
  Gain1 : Gain  Gain=1000
  Kd_pos : Constant  Value=100
  Ki_pos : Constant  Value=5
  Ki_spd : Constant  Value=700
  Kp_pos : Constant  Value=100
  Kp_spd : Constant  Value=800
  Memory : Memory
  Memory1 : Memory
  Motor Torque : Scope
  Mux : Mux
  Mux1 : Mux  Inputs=5
  Mux2 : Mux  Inputs=2
  Mux3 : Mux  Inputs=2
  Mux4 : Mux  Inputs=2
  PS-Simulink Converter : nesl_utility/PS-Simulink Converter  PhysicalDomain=network_engine_domain  SubClassName=ps_output  LeftPortType=input  RightPortType=output  PseudoPeriodic=off  Frequencies=[]  VectorFormat=inherit  Unit=inherit  AffineConversion=off
  PS-Simulink Converter1 : nesl_utility/PS-Simulink Converter  PhysicalDomain=network_engine_domain  SubClassName=ps_output  LeftPortType=input  RightPortType=output  PseudoPeriodic=off  Frequencies=[]  VectorFormat=inherit  Unit=inherit  AffineConversion=off
  Position and Speed : Scope  NumInputPorts=2
  PulleyMotor : sm_lib/Joints/Revolute Joint  JointMode=Normal  SenseConstraintForce=off  SenseConstraintForceX=off  SenseConstraintForceY=off  SenseConstraintForceZ=off  SenseConstraintTorque=off  SenseConstraintTorqueX=off  SenseConstraintTorqueY=off  SenseConstraintTorqueZ=off  SenseTotalForce=off  SenseTotalForceX=off  SenseTotalForceY=off  SenseTotalForceZ=off  SenseTotalTorque=off  SenseTotalTorqueX=off  SenseTotalTorqueY=off  SenseTotalTorqueZ=off  CompositeWrenchDir=FollowerOnBase  CompositeWrenchFrame=BaseFrame  EquilibriumPosition=0  EquilibriumPositionUnits=rad  SpringStiffness=0  SpringStiffnessUnits=N*m/rad  DampingCoefficient=0  DampingCoefficientUnits=N*m/(rad/s)  TorqueActuationMode=InputTorque  MotionActuationMode=ComputedMotion  SensePosition=on  SenseVelocity=on  SenseAcceleration=off  SenseTorqueForce=off  SenseLowerLimitTorqueForce=off  SenseUpperLimitTorqueForce=off  LowerLimitSpecify=off  LowerLimitBound=-90  LowerLimitBoundUnits=deg  LowerLimitStiffness=1e4  LowerLimitStiffnessUnits=N*m/deg  LowerLimitDamping=10  LowerLimitDampingUnits=N*m/(deg/s)  LowerLimitTransitionRegionWidth=0.1  LowerLimitTransitionRegionWidthUnits=deg  UpperLimitSpecify=off  UpperLimitBound=90  UpperLimitBoundUnits=deg  UpperLimitStiffness=1e4  UpperLimitStiffnessUnits=N*m/deg  UpperLimitDamping=10  UpperLimitDampingUnits=N*m/(deg/s)  UpperLimitTransitionRegionWidth=0.1  UpperLimitTransitionRegionWidthUnits=deg  PositionTargetSpecify=off  PositionTargetPriority=Low  PositionTargetValue=0  PositionTargetValueUnits=deg  VelocityTargetSpecify=off  VelocityTargetPriority=High  VelocityTargetValue=0  VelocityTargetValueUnits=deg/s
  PulleySubAssembly1 : Subsystem
      mask Display: image(fullfile('ElevatorSupport','Images','CabinPulley.png'));
  PulleySubAssembly2 : Subsystem
      mask Display: image(fullfile('ElevatorSupport','Images','CounterWeightPulley.png'));
  Revolute : sm_lib/Joints/Revolute Joint  JointMode=Normal  SenseConstraintForce=off  SenseConstraintForceX=off  SenseConstraintForceY=off  SenseConstraintForceZ=off  SenseConstraintTorque=off  SenseConstraintTorqueX=off  SenseConstraintTorqueY=off  SenseConstraintTorqueZ=off  SenseTotalForce=off  SenseTotalForceX=off  SenseTotalForceY=off  SenseTotalForceZ=off  SenseTotalTorque=off  SenseTotalTorqueX=off  SenseTotalTorqueY=off  SenseTotalTorqueZ=off  CompositeWrenchDir=FollowerOnBase  CompositeWrenchFrame=BaseFrame  EquilibriumPosition=0  EquilibriumPositionUnits=rad  SpringStiffness=0  SpringStiffnessUnits=N*m/rad  DampingCoefficient=0  DampingCoefficientUnits=N*m/(rad/s)  TorqueActuationMode=NoTorque  MotionActuationMode=ComputedMotion  SensePosition=off  SenseVelocity=off  SenseAcceleration=off  SenseTorqueForce=off  SenseLowerLimitTorqueForce=off  SenseUpperLimitTorqueForce=off  LowerLimitSpecify=off  LowerLimitBound=-90  LowerLimitBoundUnits=deg  LowerLimitStiffness=1e4  LowerLimitStiffnessUnits=N*m/deg  LowerLimitDamping=10  LowerLimitDampingUnits=N*m/(deg/s)  LowerLimitTransitionRegionWidth=0.1  LowerLimitTransitionRegionWidthUnits=deg  UpperLimitSpecify=off  UpperLimitBound=90  UpperLimitBoundUnits=deg  UpperLimitStiffness=1e4  UpperLimitStiffnessUnits=N*m/deg  UpperLimitDamping=10  UpperLimitDampingUnits=N*m/(deg/s)  UpperLimitTransitionRegionWidth=0.1  UpperLimitTransitionRegionWidthUnits=deg  PositionTargetSpecify=on  PositionTargetPriority=Low  PositionTargetValue=RevoluteJoint(1).Rz.Pos  PositionTargetValueUnits=deg  VelocityTargetSpecify=off  VelocityTargetPriority=High  VelocityTargetValue=1000  VelocityTargetValueUnits=deg/s
  Revolute2 : sm_lib/Joints/Revolute Joint  JointMode=Normal  SenseConstraintForce=off  SenseConstraintForceX=off  SenseConstraintForceY=off  SenseConstraintForceZ=off  SenseConstraintTorque=off  SenseConstraintTorqueX=off  SenseConstraintTorqueY=off  SenseConstraintTorqueZ=off  SenseTotalForce=off  SenseTotalForceX=off  SenseTotalForceY=off  SenseTotalForceZ=off  SenseTotalTorque=off  SenseTotalTorqueX=off  SenseTotalTorqueY=off  SenseTotalTorqueZ=off  CompositeWrenchDir=FollowerOnBase  CompositeWrenchFrame=BaseFrame  EquilibriumPosition=0  EquilibriumPositionUnits=rad  SpringStiffness=0  SpringStiffnessUnits=N*m/rad  DampingCoefficient=0  DampingCoefficientUnits=N*m/(rad/s)  TorqueActuationMode=NoTorque  MotionActuationMode=ComputedMotion  SensePosition=off  SenseVelocity=off  SenseAcceleration=off  SenseTorqueForce=off  SenseLowerLimitTorqueForce=off  SenseUpperLimitTorqueForce=off  LowerLimitSpecify=off  LowerLimitBound=-90  LowerLimitBoundUnits=deg  LowerLimitStiffness=1e4  LowerLimitStiffnessUnits=N*m/deg  LowerLimitDamping=10  LowerLimitDampingUnits=N*m/(deg/s)  LowerLimitTransitionRegionWidth=0.1  LowerLimitTransitionRegionWidthUnits=deg  UpperLimitSpecify=off  UpperLimitBound=90  UpperLimitBoundUnits=deg  UpperLimitStiffness=1e4  UpperLimitStiffnessUnits=N*m/deg  UpperLimitDamping=10  UpperLimitDampingUnits=N*m/(deg/s)  UpperLimitTransitionRegionWidth=0.1  UpperLimitTransitionRegionWidthUnits=deg  PositionTargetSpecify=on  PositionTargetPriority=Low  PositionTargetValue=RevoluteJoint(3).Rz.Pos  PositionTargetValueUnits=deg  VelocityTargetSpecify=off  VelocityTargetPriority=High  VelocityTargetValue=0  VelocityTargetValueUnits=deg/s
  Revolute3 : sm_lib/Joints/Revolute Joint  JointMode=Normal  SenseConstraintForce=off  SenseConstraintForceX=off  SenseConstraintForceY=off  SenseConstraintForceZ=off  SenseConstraintTorque=off  SenseConstraintTorqueX=off  SenseConstraintTorqueY=off  SenseConstraintTorqueZ=off  SenseTotalForce=off  SenseTotalForceX=off  SenseTotalForceY=off  SenseTotalForceZ=off  SenseTotalTorque=off  SenseTotalTorqueX=off  SenseTotalTorqueY=off  SenseTotalTorqueZ=off  CompositeWrenchDir=FollowerOnBase  CompositeWrenchFrame=BaseFrame  EquilibriumPosition=0  EquilibriumPositionUnits=rad  SpringStiffness=0  SpringStiffnessUnits=N*m/rad  DampingCoefficient=0  DampingCoefficientUnits=N*m/(rad/s)  TorqueActuationMode=NoTorque  MotionActuationMode=ComputedMotion  SensePosition=off  SenseVelocity=off  SenseAcceleration=off  SenseTorqueForce=off  SenseLowerLimitTorqueForce=off  SenseUpperLimitTorqueForce=off  LowerLimitSpecify=off  LowerLimitBound=-90  LowerLimitBoundUnits=deg  LowerLimitStiffness=1e4  LowerLimitStiffnessUnits=N*m/deg  LowerLimitDamping=10  LowerLimitDampingUnits=N*m/(deg/s)  LowerLimitTransitionRegionWidth=0.1  LowerLimitTransitionRegionWidthUnits=deg  UpperLimitSpecify=off  UpperLimitBound=90  UpperLimitBoundUnits=deg  UpperLimitStiffness=1e4  UpperLimitStiffnessUnits=N*m/deg  UpperLimitDamping=10  UpperLimitDampingUnits=N*m/(deg/s)  UpperLimitTransitionRegionWidth=0.1  UpperLimitTransitionRegionWidthUnits=deg  PositionTargetSpecify=on  PositionTargetPriority=Low  PositionTargetValue=RevoluteJoint(4).Rz.Pos  PositionTargetValueUnits=deg  VelocityTargetSpecify=off  VelocityTargetPriority=High  VelocityTargetValue=0  VelocityTargetValueUnits=deg/s
  RoofTop_1_RIGID : Subsystem
      mask Display: image(fullfile('ElevatorSupport','Images','Roof.png'));
  S-Function : S-Function  FunctionName=SPD_CTRL  SFunctionDeploymentMode=off  EnableBusSupport=off
  S-Function1 : S-Function  FunctionName=POS_CTRL  SFunctionDeploymentMode=off  EnableBusSupport=off
  S-Function2 : S-Function  FunctionName=DCMotor  SFunctionDeploymentMode=off  EnableBusSupport=off
  Simulink-PS Converter : nesl_utility/Simulink-PS Converter  PhysicalDomain=network_engine_domain  SubClassName=ps_input  LeftPortType=input  RightPortType=output  PseudoPeriodic=off  Frequencies=[]  NoiseDistribution=none  NoiseParameters=[]  Unit=1  AffineConversion=off  FilteringAndDerivatives=provide  SimscapeFilterOrder=1  InputFilterTimeConstant=0.001  UdotUserProvided=0
  shaft1 : Subsystem
  shaft2 : Subsystem
  E1 : PMIOPort  Side=Right
  CW1 : PMIOPort  Port=2  Side=Right
  CW2 : PMIOPort  Port=3  Side=Right
  CW4 : PMIOPort  Port=4  Side=Right
  CW5 : PMIOPort  Port=5  Side=Right
  CW3 : PMIOPort  Port=6  Side=Right
  B : PMIOPort  Port=7  Side=Left
  E2 : PMIOPort  Port=8  Side=Right
  E3 : PMIOPort  Port=9  Side=Right
  E4 : PMIOPort  Port=10  Side=Right
  E5 : PMIOPort  Port=11  Side=Right
  wires:
  Mux/1 -> S-Function/1
  Kp_spd/1 -> Mux/1
  Ki_spd/1 -> Mux/2
  PS-Simulink Converter/1 -> Mux3/2, Memory/1, Mux2/2  "w_act"
  Memory/1 -> Mux/4  "w_act"
  S-Function1/1 -> Mux3/1, Mux/3  "w_ref"
  Add Constant/1 -> Motor Torque/1, Simulink-PS Converter/1
  Mux1/1 -> S-Function1/1
  PS-Simulink Converter1/1 -> Memory1/1  "pos_act"
  Ki_pos/1 -> Mux1/2
  Kp_pos/1 -> Mux1/1
  Memory1/1 -> Mux4/2, Mux1/5  "pos_act"
  Motor_In/1 -> Mux4/1, Mux1/4  "pos_ref"
  S-Function/1 -> Mux2/1
  Mux2/1 -> S-Function2/1
  S-Function2/1 -> Gain1/1
  Gain1/1 -> Add Constant/1
  Kd_pos/1 -> Mux1/3
  Mux4/1 -> Position and Speed/1
  Mux3/1 -> Position and Speed/2
  connections:
  PulleySubAssembly1/RConn2 -- PulleySubAssembly2/RConn2
  Revolute3/LConn1 -- RoofTop_1_RIGID/RConn1
  PulleySubAssembly1/RConn4 -- PulleySubAssembly2/RConn4
  PulleySubAssembly1/RConn8 -- PulleySubAssembly2/RConn8
  PulleySubAssembly1/LConn1 -- Revolute/RConn1
  PulleySubAssembly1/RConn6 -- PulleySubAssembly2/RConn6
  Revolute/LConn1 -- RoofTop_1_RIGID/RConn4
  PulleySubAssembly1/RConn1 -- E1/RConn1
  PulleyMotor/LConn1 -- RoofTop_1_RIGID/RConn3
  PulleySubAssembly1/RConn5 -- E3/RConn1
  PulleySubAssembly1/RConn3 -- E2/RConn1
  Revolute3/RConn1 -- shaft1/LConn1
  B/RConn1 -- RoofTop_1_RIGID/LConn1
  Revolute2/LConn1 -- RoofTop_1_RIGID/RConn2
  PulleySubAssembly1/RConn7 -- E4/RConn1
  Revolute2/RConn1 -- shaft2/LConn1
  PulleySubAssembly2/RConn10 -- PulleySubAssembly1/RConn10
  CW4/RConn1 -- PulleySubAssembly2/RConn7
  PulleySubAssembly2/LConn1 -- PulleyMotor/RConn1
  PulleySubAssembly2/RConn9 -- CW5/RConn1
  PulleySubAssembly1/RConn9 -- E5/RConn1
  PulleySubAssembly2/RConn1 -- CW1/RConn1
  CW2/RConn1 -- PulleySubAssembly2/RConn3
  PulleySubAssembly2/RConn5 -- CW3/RConn1
  PulleyMotor/LConn2 -- Simulink-PS Converter/RConn1
  PulleyMotor/RConn3 -- PS-Simulink Converter/LConn1
  PS-Simulink Converter1/LConn1 -- PulleyMotor/RConn2

== system Elevator/Elevator Floor Input/FloorChangesStairSignal ==
  In1 : Inport
  1-D Lookup Table : Lookup_n-D  NumberOfTableDimensions=1  BreakpointsForDimension1=FloorTimeStairOut  BreakpointsForDimension1FirstPoint=2  Table=FloorStairOut  ExtrapMethod=Clip  UseLastTableValue=on  InternalRulePriority=Speed  RndMeth=Nearest
  1-D Lookup Table1 : Lookup_n-D  NumberOfTableDimensions=1  BreakpointsForDimension1=StairOutTime2  BreakpointsForDimension1FirstPoint=2  Table=StairOutTime1  ExtrapMethod=Clip  UseLastTableValue=on  InternalRulePriority=Speed  RndMeth=Nearest
  1-D Lookup Table2 : Lookup_n-D  NumberOfTableDimensions=1  BreakpointsForDimension1=DoorStairOutTime2  BreakpointsForDimension1FirstPoint=2  Table=DoorStairOutTime1  ExtrapMethod=Clip  UseLastTableValue=on  InternalRulePriority=Speed  RndMeth=Nearest
  FloorChanges : Outport  VectorParamsAs1DForOutWhenUnconnected=off
  TimeChanges : Outport  Port=2  VectorParamsAs1DForOutWhenUnconnected=off
  DoorTimeChanges : Outport  Port=3  VectorParamsAs1DForOutWhenUnconnected=off
  wires:
  In1/1 -> 1-D Lookup Table2/1, 1-D Lookup Table1/1, 1-D Lookup Table/1
  1-D Lookup Table/1 -> FloorChanges/1
  1-D Lookup Table1/1 -> TimeChanges/1
  1-D Lookup Table2/1 -> DoorTimeChanges/1

== system Elevator/Elevator Assembly/Building/Floors ==
  Base : Subsystem
  Floor0 : Subsystem
  Floor1 : Subsystem
  Floor2 : Subsystem
  Floor3 : Subsystem
  Floor4 : Subsystem
  Floor5 : Subsystem
  Floor6 : Subsystem
  Floor7 : Subsystem
  Conn1 : PMIOPort  Side=Left
  Conn2 : PMIOPort  Port=2  Side=Right
  connections:
  Floor1/LConn1 -- Floor0/LConn1
  Floor7/LConn1 -- Floor6/LConn2
  Floor7/LConn2 -- Conn1/RConn1
  Floor5/LConn2 -- Floor6/LConn1
  Floor7/LConn3 -- Conn2/RConn1
  Floor2/LConn1 -- Floor1/LConn2
  Floor3/LConn1 -- Floor2/LConn2
  Floor4/LConn1 -- Floor3/LConn2
  Floor5/LConn1 -- Floor4/LConn2
  Base/LConn1 -- Floor0/RConn1

== system Elevator/Elevator Assembly/Building/LongRail_1_RIGID ==
  ReferenceFrame : sm_lib/Frames and Transforms/Reference Frame
  Solid : sm_lib/Body Elements/File Solid  ExtGeomFileName=CouterWeightRail.step  UnitType=FromFile  ExtGeomFileUnits=m  StepReaderType=HEX  ExportConvexHullGeometry=off  InertiaType=Custom  Mass=CouterWeightRail.mass  MassUnits=kg  CenterOfMass=CouterWeightRail.CoM  CenterOfMassUnits=mm  MomentsOfInertia=CouterWeightRail.MoI  MomentsOfInertiaUnits=kg*mm^2  ProductsOfInertia=CouterWeightRail.PoI  ProductsOfInertiaUnits=kg*mm^2  BasedOnType=DensityFromFile  Density=1000  DensityUnits=kg/m^3  DoExposeReferenceFrame=on  SerializedFrames=<Frames/>  GraphicType=FromGeometry  MarkerShape=Sphere  MarkerSize=10  GraphicVisPropType=SimpleVisualProperties  GraphicDiffuseColor=[0.0 0.0 0.0]  GraphicSpecularColor=[0.5 0.5 0.5 1.0]  GraphicAmbientColor=[0.15 0.15 0.15 1.0]  GraphicEmissiveColor=[0.0 0.0 0.0 1.0]  GraphicShininess=75  GraphicOpacity=1
  Transform : sm_lib/Frames and Transforms/Rigid Transform  TranslationMethod=Cartesian  TranslationStandardOffset=0  TranslationStandardOffsetUnits=mm  TranslationStandardAxis=+Z  TranslationCartesianOffset=RigidTransform(1).translation  TranslationCartesianOffsetUnits=mm  TranslationROffset=0  TranslationROffsetUnits=m  TranslationZOffset=0  TranslationZOffsetUnits=m  TranslationThetaOffset=0  TranslationThetaOffsetUnits=deg  RotationMethod=ArbitraryAxis  RotationAngleUnits=rad  RotationStandardAxis=+Z  RotationAngle=RigidTransform(1).angle  RotationArbitraryAxis=RigidTransform(1).axis  FollAlignAxisA=+X  BaseAlignAxisA=+Y  FollAlignAxisB=+Y  BaseAlignAxisB=+Z  RotationSequenceAxes=FollowerAxes  RotationSequence=XYX  RotationSequenceAngles=[0 0 0]  RotationSequenceAnglesUnits=deg  RotationMatrix=[1 0 0; 0 1 0; 0 0 1]  Quaternion=[1 0 0 0]
  Transform1 : sm_lib/Frames and Transforms/Rigid Transform  TranslationMethod=Cartesian  TranslationStandardOffset=0  TranslationStandardOffsetUnits=mm  TranslationStandardAxis=+Z  TranslationCartesianOffset=RigidTransform(4).translation  TranslationCartesianOffsetUnits=mm  TranslationROffset=0  TranslationROffsetUnits=m  TranslationZOffset=0  TranslationZOffsetUnits=m  TranslationThetaOffset=0  TranslationThetaOffsetUnits=deg  RotationMethod=ArbitraryAxis  RotationAngleUnits=rad  RotationStandardAxis=+Z  RotationAngle=RigidTransform(4).angle  RotationArbitraryAxis=RigidTransform(4).axis  FollAlignAxisA=+X  BaseAlignAxisA=+Y  FollAlignAxisB=+Y  BaseAlignAxisB=+Z  RotationSequenceAxes=FollowerAxes  RotationSequence=XYX  RotationSequenceAngles=[0 0 0]  RotationSequenceAnglesUnits=deg  RotationMatrix=[1 0 0; 0 1 0; 0 0 1]  Quaternion=[1 0 0 0]
  Transform2 : sm_lib/Frames and Transforms/Rigid Transform  TranslationMethod=Cartesian  TranslationStandardOffset=0  TranslationStandardOffsetUnits=mm  TranslationStandardAxis=+Z  TranslationCartesianOffset=RigidTransform(18).translation  TranslationCartesianOffsetUnits=mm  TranslationROffset=0  TranslationROffsetUnits=m  TranslationZOffset=0  TranslationZOffsetUnits=m  TranslationThetaOffset=0  TranslationThetaOffsetUnits=deg  RotationMethod=ArbitraryAxis  RotationAngleUnits=rad  RotationStandardAxis=+Z  RotationAngle=RigidTransform(18).angle  RotationArbitraryAxis=RigidTransform(18).axis  FollAlignAxisA=+X  BaseAlignAxisA=+Y  FollAlignAxisB=+Y  BaseAlignAxisB=+Z  RotationSequenceAxes=FollowerAxes  RotationSequence=XYX  RotationSequenceAngles=[0 0 0]  RotationSequenceAnglesUnits=deg  RotationMatrix=[1 0 0; 0 1 0; 0 0 1]  Quaternion=[1 0 0 0]
  F1 : PMIOPort  Side=Left
  F : PMIOPort  Port=2  Side=Left
  F2 : PMIOPort  Port=3  Side=Left
  connections:
  ReferenceFrame/RConn1 -- Transform1/LConn1 -- Transform2/LConn1 -- Solid/RConn1 -- Transform/LConn1
  Transform/RConn1 -- F/RConn1
  Transform1/RConn1 -- F1/RConn1
  Transform2/RConn1 -- F2/RConn1
